simulink model "QuadrotorSimCircle"  (R2023b)
settings: Solver=FixedStepAuto  StartTime=0.0  StopTime=150  FixedStep=0.001  RelTol=1e-3
undefined symbols (not defined in the file or in its folder): magnitude
libraries: aerolibutil x1
settings Model: Creator=kevin  LastModifiedBy=kevin

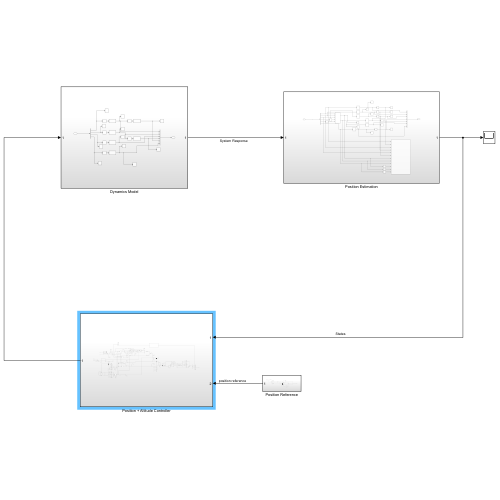
[thumbnail: Simulink's stored preview of the top-level diagram]
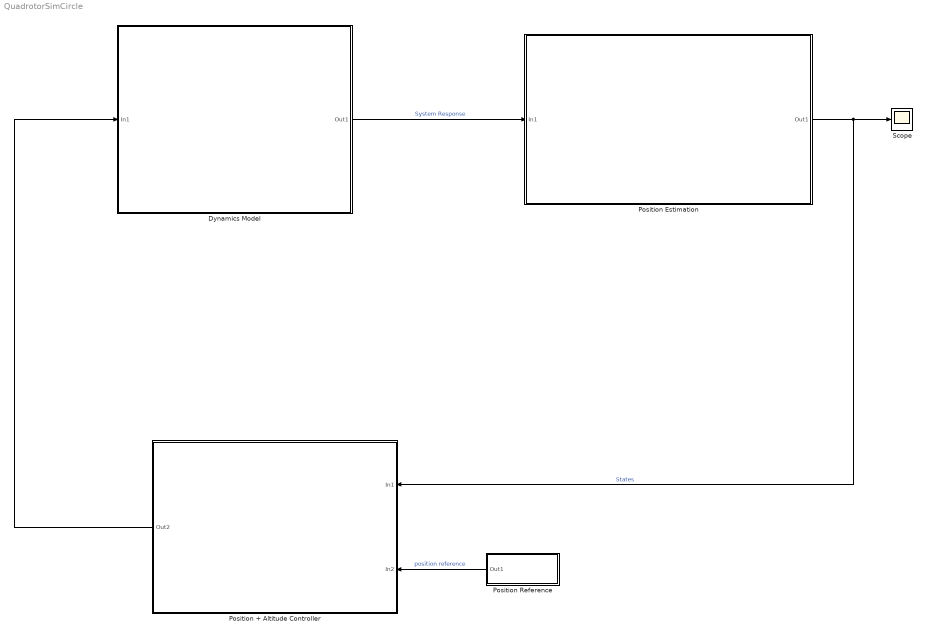
== system QuadrotorSimCircle ==
  Dynamics Model : Subsystem
  Position + Altitude Controller : Subsystem
  Position Estimation : Subsystem
  Position Reference : Subsystem
  Scope : Scope
  wires:
  Dynamics Model/1(Out1) -> Position Estimation/1(In1)  "System Response"
  Position Reference/1(Out1) -> Position + Altitude Controller/2(In2)  "position reference"
  Position Estimation/1(Out1) -> Position + Altitude Controller/1(In1), Scope/1  "States"
  Position + Altitude Controller/1(Out2) -> Dynamics Model/1(In1)

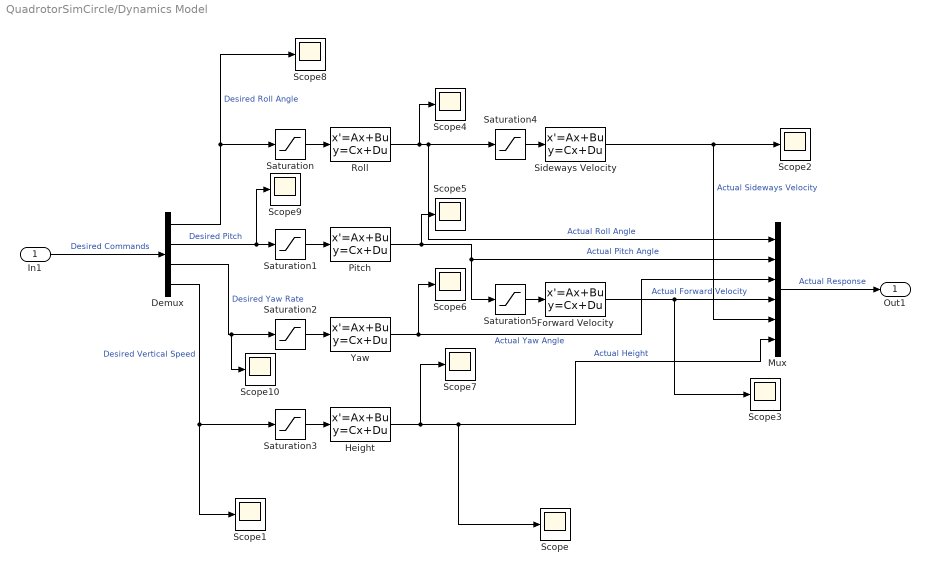
== system QuadrotorSimCircle/Dynamics Model ==
  In1 : Inport
  Demux : Demux
  Forward Velocity : StateSpace  A=[-0.4596]  B=[2]  C=[2.3868]  D=[0]  InitialCondition=0
  Height : StateSpace  A=[-5.8200, -0.0000036046; 0.0000038147, 0]  B=[1024; 0]  C=[0.00014907, 1319.1]  D=[0]  InitialCondition=0
  Mux : Mux  Inputs=6
  Pitch : StateSpace  A=[-3.9784, -2.9796; 4, 0]  B=[2;0]  C=[1.2569, 0.6083]  D=[0]  InitialCondition=0
  Roll : StateSpace  A=[-4.2683, -3.1716; 4, 0]  B=[2;0]  C=[0.7417, 0.4405]  D=[0]  InitialCondition=0
  Saturation{,1..5} (6 alike) : Saturate  UpperLimit=1  LowerLimit=-1
  Scope{,1..10} (11 alike) : Scope
  Sideways Velocity : StateSpace  A=[-0.4596]  B=[2]  C=[2.3868]  D=[0]  InitialCondition=0
  Yaw : StateSpace  A=[-0.0059]  B=[1]  C=[1.2653]  D=[0]  InitialCondition=0
  Out1 : Outport
  wires:
  Demux/2 -> Scope9/1, Saturation1/1  "Desired Pitch"
  Demux/3 -> Scope10/1, Saturation2/1  "Desired Yaw Rate"
  Demux/4 -> Scope1/1, Saturation3/1  "Desired Vertical Speed"
  Pitch/1 -> Scope5/1, Saturation5/1, Mux/2  "Actual Pitch Angle"
  Forward Velocity/1 -> Scope3/1, Mux/4  "Actual Forward Velocity"
  Roll/1 -> Mux/1, Saturation4/1, Scope4/1  "Actual Roll Angle"
  Sideways Velocity/1 -> Mux/5, Scope2/1  "Actual Sideways Velocity"
  Mux/1 -> Out1/1  "Actual Response"
  Yaw/1 -> Scope6/1, Mux/3  "Actual Yaw Angle"
  In1/1 -> Demux/1  "Desired Commands"
  Demux/1 -> Scope8/1, Saturation/1  "Desired Roll Angle"
  Height/1 -> Scope7/1, Mux/6, Scope/1  "Actual Height"
  Saturation/1 -> Roll/1
  Saturation1/1 -> Pitch/1
  Saturation2/1 -> Yaw/1
  Saturation3/1 -> Height/1
  Saturation4/1 -> Sideways Velocity/1
  Saturation5/1 -> Forward Velocity/1

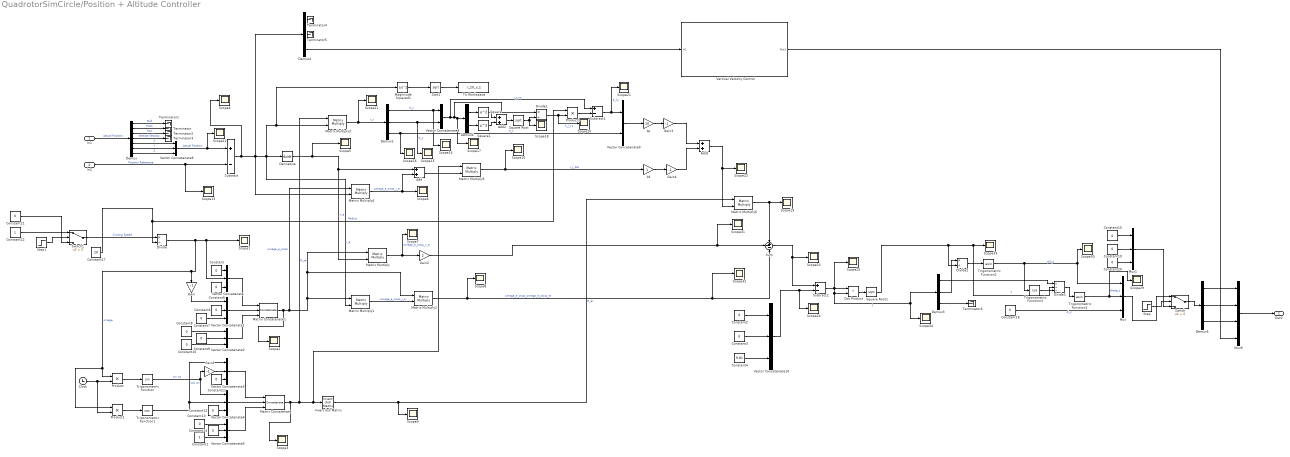
== system QuadrotorSimCircle/Position + Altitude Controller ==
  In1 : Inport
  In2 : Inport  Port=2
  Add : Sum
  Add1 : Sum
  Add2 : Sum
  Clock : Clock
  Constant{,2..3,5..15,18..21} (18 alike) : Constant  Value=0
  Constant1 : Constant
  Constant17 : Constant  Value=20
  Constant22 : Constant
  Constant4 : Constant  Value=9.81
  Demux : Demux  Outputs=7
  Demux{1..3,5} (4 alike) : Demux  Outputs=3
  Demux4 : Demux  Outputs=2
  Derivative : Derivative
  Divide : Product  Inputs=*/
  Divide1 : Product  Inputs=*/
  Divide2 : Product  Inputs=*/
  Divide3 : Product  Inputs=*//
  Dot Product : DotProduct  OutDataTypeStr=Inherit: Inherit via internal rule
  Gain{,1,3..4} (4 alike) : Gain  Gain=-1
  Gain2 : Gain  Gain=2
  Invert 3x3 Matrix : aerolibutil/Invert  3x3 Matrix
  Magnitude Squared1 : Math  Operator=magnitude^2
  Matrix Concatenate : Concatenate  NumInputs=3  Mode=Multidimensional array  ConcatenateDimension=2
  Matrix Concatenate1 : Concatenate  NumInputs=3  Mode=Multidimensional array  ConcatenateDimension=2
  Matrix Multiply{,1..6} (7 alike) : Product  Multiplication=Matrix(*)
  Mux : Mux  Inputs=3
  Mux1 : Mux  Inputs=3
  Mux9 : Mux
  Product : Product
  Product1 : Product
  Product3 : Product
  Scope{1..25,29..34} (31 alike) : Scope
  Sqrt1 : Sqrt
  Square : Math  Operator=square
  Square Root : Sqrt
  Square Root1 : Sqrt
  Square1 : Math  Operator=square
  Step : Step  Time=10  SampleTime=0
  Step1 : Step  Time=10  SampleTime=0
  Subtract : Sum  Inputs=+-
  Subtract1 : Sum  Inputs=+-
  Subtract2 : Sum  Inputs=+-
  Sum : Sum  Inputs=+--
  Switch : Switch  Criteria=u2 > Threshold  SaturateOnIntegerOverflow=off  InputSameDT=off
  Switch1 : Switch  Criteria=u2 > Threshold  SaturateOnIntegerOverflow=off  InputSameDT=off
  Terminator{,1..6} (7 alike) : Terminator
  To Workspace : ToWorkspace  VariableName=r_20_v_1  SampleTime=-1
  Trigonometric Function : Trigonometry
  Trigonometric Function1 : Trigonometry  Operator=cos
  Trigonometric Function2 : Trigonometry  Operator=asin
  Trigonometric Function3 : Trigonometry  Operator=cos
  Trigonometric Function4 : Trigonometry  Operator=asin
  Vector Concatenate{,1..6,10} (8 alike) : Concatenate  NumInputs=3
  Vector Concatenate8 : Concatenate
  Vector Concatenate9 : Concatenate
  Vertical Velocity Control : Subsystem
  kd : Gain
  kp : Gain  Gain=10
  Out2 : Outport
  wires:
  In1/1 -> Demux/1  "Actual Position"
  In2/1 -> Scope13/1, Subtract/2  "Position Reference"
  Demux/1 -> Terminator1/1  "Roll"
  Demux/2 -> Terminator/1  "Pitch"
  Demux/3 -> Terminator2/1  "Yaw"
  Demux/4 -> Terminator3/1  "Vertical Velocity"
  Demux/5 -> Vector Concatenate6/1  "X"
  Demux/6 -> Vector Concatenate6/2  "Y"
  Demux/7 -> Vector Concatenate6/3  "Z"
  Switch1/1 -> Divide/1  "Crusing Speed"
  Constant17/1 -> Divide/2, Product3/1  "Radius"
  Vector Concatenate/1 -> Matrix Concatenate1/1
  Vector Concatenate1/1 -> Matrix Concatenate1/2
  Vector Concatenate2/1 -> Matrix Concatenate1/3
  Matrix Concatenate1/1 -> Scope2/1, Matrix Multiply4/1, Matrix Multiply1/1, Matrix Multiply/1, Matrix Multiply2/1  "omega_e_cross"
  Vector Concatenate5/1 -> Matrix Concatenate/3
  Vector Concatenate4/1 -> Matrix Concatenate/2
  Vector Concatenate3/1 -> Matrix Concatenate/1
  Clock/1 -> Product1/2, Product/2
  Product/1 -> Trigonometric Function/1
  Trigonometric Function/1 -> Vector Concatenate4/1, Gain1/1  "sin wt"
  Product1/1 -> Trigonometric Function1/1
  Trigonometric Function1/1 -> Vector Concatenate4/2, Vector Concatenate3/1  "cos wt"
  Constant1/1 -> Vector Concatenate5/3
  Matrix Concatenate/1 -> Scope3/1, Matrix Multiply3/1, Invert 3x3 Matrix/1, Matrix Multiply5/1  "R_re"
  Vector Concatenate6/1 -> Subtract/1, Scope12/1  "Actual Position"
  Subtract/1 -> Scope4/1, Demux2/1, Matrix Multiply1/2, Derivative/1, Magnitude Squared1/1, Matrix Multiply3/2, Matrix Multiply4/2  "r_e"
  Invert 3x3 Matrix/1 -> Scope9/1, Matrix Multiply6/1  "R_er"
  Derivative/1 -> Scope5/1, Add/1, Matrix Multiply/2  "v_e"
  Matrix Multiply/1 -> Scope7/1, Gain2/1  "omega_e_cross_v_e"
  Gain2/1 -> Scope31/1, Sum/2
  Matrix Multiply1/1 -> Matrix Multiply2/2  "omega_e_cross_r_e"
  Matrix Multiply2/1 -> Scope8/1, Scope32/1, Sum/3  "omega_e_cross_omega_e_cross_re"
  Matrix Multiply3/1 -> Scope11/1, Demux1/1  "r_r"
  Demux1/1 -> Vector Concatenate8/1, Scope14/1  "e_x"
  Demux1/2 -> Vector Concatenate8/2, Scope15/1  "e_y"
  Demux1/3 -> Scope16/1, Vector Concatenate9/2  "e_z"
  Vector Concatenate8/1 -> Subtract1/1, Divide1/1, Scope17/1, Demux4/1  "r_r_xy"
  Divide1/1 -> Scope20/1, Product3/2  "n_r_xy"
  Product3/1 -> Subtract1/2
  Subtract1/1 -> Scope21/1, Vector Concatenate9/1  "e_xy"
  Matrix Multiply4/1 -> Scope6/1, Add/2  "omega_e_cross_r_e"
  Add/1 -> Matrix Multiply5/2
  Matrix Multiply5/1 -> Scope10/1, kd/1  "r_r_dot"
  Vector Concatenate9/1 -> kp/1
  kp/1 -> Gain3/1
  kd/1 -> Gain4/1
  Add1/1 -> Scope22/1, Matrix Multiply6/2
  Sum/1 -> Scope23/1, Subtract2/1
  Constant2/1 -> Vector Concatenate10/1
  Constant3/1 -> Vector Concatenate10/2
  Constant4/1 -> Vector Concatenate10/3
  Vector Concatenate10/1 -> Scope24/1, Subtract2/2
  Constant/1 -> Vector Concatenate/1
  Constant5/1 -> Vector Concatenate/3
  Constant6/1 -> Vector Concatenate1/2
  Constant7/1 -> Vector Concatenate1/3
  Constant8/1 -> Vector Concatenate2/1
  Constant9/1 -> Vector Concatenate2/2
  Constant10/1 -> Vector Concatenate2/3
  Constant11/1 -> Vector Concatenate3/3
  Constant12/1 -> Vector Concatenate4/3
  Constant13/1 -> Vector Concatenate5/1
  Constant14/1 -> Vector Concatenate5/2
  Magnitude Squared1/1 -> Sqrt1/1
  Sqrt1/1 -> To Workspace/1
  Divide/1 -> Vector Concatenate/2, Scope1/1, Gain/1, Product1/1, Product/1  "omega"
  Mux9/1 -> Out2/1
  Trigonometric Function2/1 -> Trigonometric Function3/1, Mux/1, Scope30/1  "phi_c"
  Demux3/1 -> Divide3/1
  Subtract2/1 -> Demux3/1, Scope34/1, Dot Product/2, Scope25/1, Dot Product/1  "f"
  Constant18/1 -> Mux/3  "si_c"
  Trigonometric Function4/1 -> Mux/2, Scope29/1  "theta_c"
  Gain/1 -> Vector Concatenate1/1
  Gain1/1 -> Vector Concatenate3/2
  Demux2/3 -> Vertical Velocity Control/1(In1)
  Vertical Velocity Control/1(Out1) -> Mux9/4
  Gain3/1 -> Add1/1
  Gain4/1 -> Add1/2
  Demux4/2 -> Square1/1
  Demux4/1 -> Square/1
  Square/1 -> Add2/1
  Square1/1 -> Add2/2
  Add2/1 -> Square Root/1
  Square Root/1 -> Scope18/1, Divide1/2
  Matrix Multiply6/1 -> Sum/1, Scope19/1
  Demux3/2 -> Divide2/1
  Demux3/3 -> Terminator6/1
  Dot Product/1 -> Square Root1/1
  Square Root1/1 -> Divide3/2, Scope33/1, Divide2/2  "T"
  Step/1 -> Switch/2
  Mux/1 -> Switch/1
  Switch/1 -> Demux5/1
  Constant15/1 -> Mux1/1
  Constant19/1 -> Mux1/2
  Constant20/1 -> Mux1/3
  Mux1/1 -> Switch/3
  Demux5/1 -> Mux9/1
  Demux5/2 -> Mux9/2
  Demux5/3 -> Mux9/3
  Step1/1 -> Switch1/2
  Constant21/1 -> Switch1/3
  Constant22/1 -> Switch1/1
  Divide2/1 -> Trigonometric Function2/1
  Trigonometric Function3/1 -> Divide3/3
  Divide3/1 -> Trigonometric Function4/1

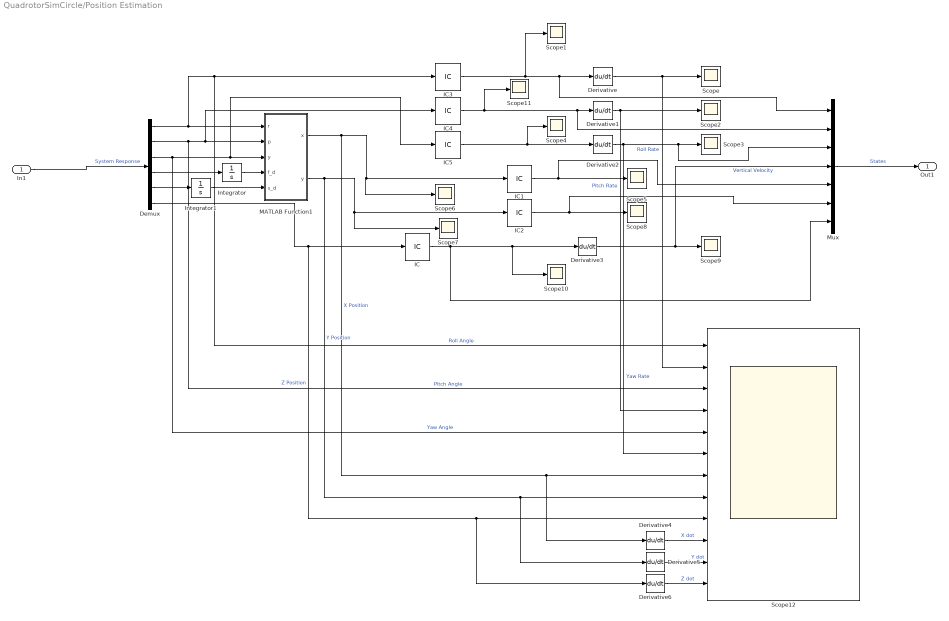
== system QuadrotorSimCircle/Position Estimation ==
  In1 : Inport
  Demux : Demux  Outputs=6
  Derivative{,1..6} (7 alike) : Derivative
  IC{,1..5} (6 alike) : InitialCondition  Value=0
  Integrator : Integrator
  Integrator1 : Integrator
  MATLAB Function1 : MATLAB Function  TreatAsAtomicUnit=on
  Mux : Mux  Inputs=7
  Scope{,1..11} (12 alike) : Scope
  Scope12 : Scope  NumInputPorts=12
  Out1 : Outport
  wires:
  In1/1 -> Demux/1  "System Response"
  Demux/1 -> Scope12/1, IC3/1, MATLAB Function1/1(r)  "Roll Angle"
  Demux/6 -> Derivative6/1, Scope12/9, IC/1  "Z Position"
  MATLAB Function1/1(x) -> Derivative4/1, Scope12/7, Scope6/1, IC1/1  "X Position"
  Demux/2 -> Scope12/3, IC4/1, MATLAB Function1/2(p)  "Pitch Angle"
  Demux/3 -> Scope12/5, IC5/1, MATLAB Function1/3("y ")  "Yaw Angle"
  Mux/1 -> Out1/1  "States"
  Derivative/1 -> Scope12/2, Scope/1  "Roll Rate"
  Derivative1/1 -> Scope2/1, Scope12/4  "Pitch Rate"
  Derivative2/1 -> Mux/3, Scope3/1, Scope12/6  "Yaw Rate"
  Derivative3/1 -> Mux/4, Scope9/1  "Vertical Velocity"
  IC/1 -> Mux/7, Scope10/1, Derivative3/1
  IC2/1 -> Mux/6, Scope8/1
  IC1/1 -> Mux/5, Scope5/1
  IC3/1 -> Scope1/1, Mux/1, Derivative/1
  IC4/1 -> Scope11/1, Mux/2, Derivative1/1
  IC5/1 -> Scope4/1, Derivative2/1
  Demux/5 -> Integrator1/1
  Demux/4 -> Integrator/1
  MATLAB Function1/2(y) -> Derivative5/1, Scope12/8, IC2/1, Scope7/1  "Y Position"
  Integrator/1 -> MATLAB Function1/4(f_d)
  Integrator1/1 -> MATLAB Function1/5(s_d)
  Derivative4/1 -> Scope12/10  "X dot"
  Derivative5/1 -> Scope12/11  "Y dot"
  Derivative6/1 -> Scope12/12  "Z dot"

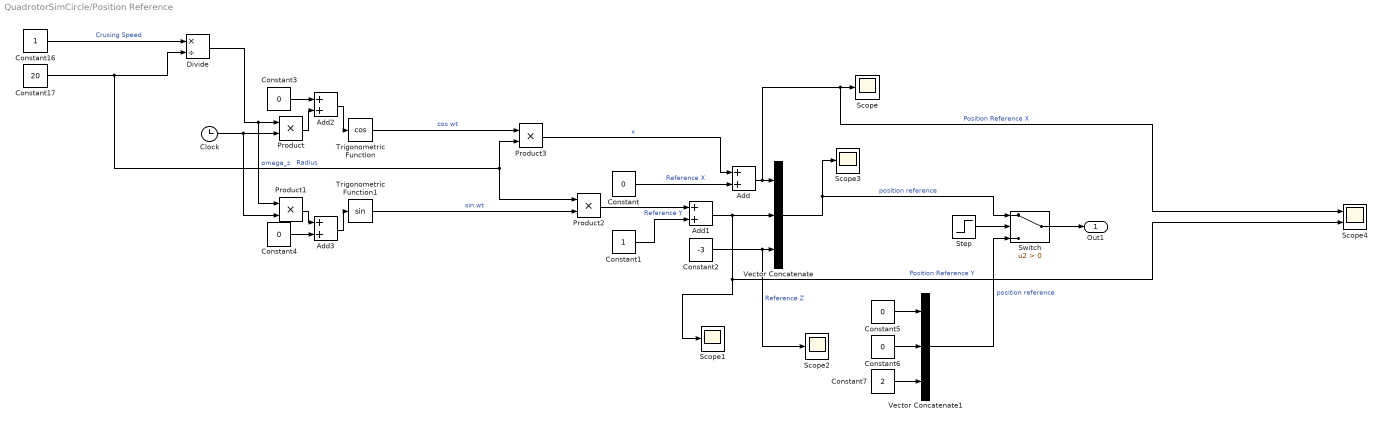
== system QuadrotorSimCircle/Position Reference ==
  Add{,1..3} (4 alike) : Sum
  Clock : Clock
  Constant{,3..6} (5 alike) : Constant  Value=0
  Constant1 : Constant
  Constant16 : Constant
  Constant17 : Constant  Value=20
  Constant2 : Constant  Value=-3
  Constant7 : Constant  Value=2
  Divide : Product  Inputs=*/
  Product{,1..3} (4 alike) : Product
  Scope{,1..3} (4 alike) : Scope
  Scope4 : Scope  NumInputPorts=2
  Step : Step  Time=10  SampleTime=0
  Switch : Switch  Criteria=u2 > Threshold  SaturateOnIntegerOverflow=off  InputSameDT=off
  Trigonometric Function : Trigonometry  Operator=cos
  Trigonometric Function1 : Trigonometry
  Vector Concatenate : Concatenate  NumInputs=3
  Vector Concatenate1 : Concatenate  NumInputs=3
  Out1 : Outport
  wires:
  Vector Concatenate/1 -> Switch/1, Scope3/1  "position reference"
  Constant/1 -> Add/2  "Reference X"
  Constant2/1 -> Vector Concatenate/3, Scope2/1  "Reference Z"
  Product1/1 -> Add3/1
  Clock/1 -> Product1/2, Product/2
  Product/1 -> Add2/2
  Constant16/1 -> Divide/1  "Crusing Speed"
  Trigonometric Function1/1 -> Product2/2  "sin wt"
  Constant17/1 -> Product2/1, Product3/2, Divide/2  "Radius"
  Product3/1 -> Add/1  "x"
  Product2/1 -> Add1/1
  Trigonometric Function/1 -> Product3/1  "cos wt"
  Add/1 -> Vector Concatenate/1, Scope4/1, Scope/1  "Position Reference X"
  Constant1/1 -> Add1/2  "Reference Y"
  Add1/1 -> Vector Concatenate/2, Scope4/2, Scope1/1  "Position Reference Y"
  Divide/1 -> Product1/1, Product/1  "omega_z"
  Add2/1 -> Trigonometric Function/1
  Add3/1 -> Trigonometric Function1/1
  Constant3/1 -> Add2/1
  Constant4/1 -> Add3/2
  Step/1 -> Switch/2
  Constant5/1 -> Vector Concatenate1/1
  Constant6/1 -> Vector Concatenate1/2
  Constant7/1 -> Vector Concatenate1/3
  Vector Concatenate1/1 -> Switch/3  "position reference"
  Switch/1 -> Out1/1

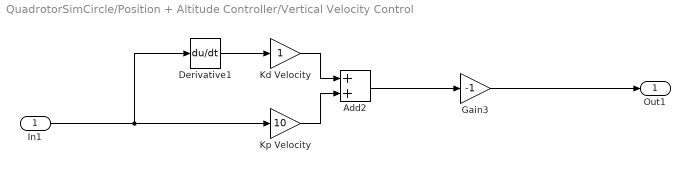
== system QuadrotorSimCircle/Position + Altitude Controller/Vertical Velocity Control ==
  In1 : Inport
  Add2 : Sum
  Derivative1 : Derivative
  Gain3 : Gain  Gain=-1
  Kd Velocity : Gain
  Kp Velocity : Gain  Gain=10
  Out1 : Outport
  wires:
  Gain3/1 -> Out1/1
  Add2/1 -> Gain3/1
  In1/1 -> Derivative1/1, Kp Velocity/1
  Kd Velocity/1 -> Add2/1
  Derivative1/1 -> Kd Velocity/1
  Kp Velocity/1 -> Add2/2

== matlab function QuadrotorSimCircle/Position Estimation/MATLAB Function1 ==
  data: r input; x output; p input; y input; f_d input; s_d input; y output
function [x, y] = fcn(r,p,y,f_d,s_d)
    Rx = [1,0,0;0,cos(r),-sin(r);0,sin(r),cos(r)];
    Ry = [cos(p),0,sin(p);0,1,0;-sin(p),0,cos(p)];
    Rz = [cos(y),-sin(y),0;sin(y),cos(y),0;0,0,1];
    R_BE = Rx*Ry*Rz;
    R_EB = R_BE.';
    d_i = R_EB*[f_d;s_d;1];
    x = d_i(1);
    y = d_i(2);
end
